simulink model "simulinkmodel"  (R2023a)
settings: Solver=ode4  StartTime=0.0  StopTime=250.0  FixedStep=1e-3  RelTol=1e-3
values from neighbouring files (symbols this model uses):
  ARw = 7.9456    [EOMs_of_AC.m]    (also in constants_simulinkmodel.m)
  b = 9.16    [EOMs_of_AC.m]    (also in constants_simulinkmodel.m)
  c = 1.3333    [EOMs_of_AC.m]    (also in constants_simulinkmodel.m)
  CDf = .005    (= 0.005)    [EOMs_of_AC.m]    (also in constants_simulinkmodel.m)
  CDmint = .002    (= 0.002)    [EOMs_of_AC.m]    (also in constants_simulinkmodel.m)
  CDminvt = .001    (= 0.001)    [EOMs_of_AC.m]    (also in constants_simulinkmodel.m)
  CDminw = .011    (= 0.011)    [EOMs_of_AC.m]    (also in constants_simulinkmodel.m)
  cgt = 3.5    [EOMs_of_AC.m]    (also in constants_simulinkmodel.m)
  cgvt = cgt    (= 3.5)    [EOMs_of_AC.m]    (also in constants_simulinkmodel.m)
  cgw = -.416    (= -0.416)    [EOMs_of_AC.m]    (also in constants_simulinkmodel.m)
  CLat = .76    (= 0.76)    [EOMs_of_AC.m]    (also in constants_simulinkmodel.m)
  CLavt = .0969    (= 0.0969)    [EOMs_of_AC.m]    (also in constants_simulinkmodel.m)
  CLaw = 4.59    [EOMs_of_AC.m]    (also in constants_simulinkmodel.m)
  Clb = -.1    (= -0.1)    [EOMs_of_AC.m]    (also in constants_simulinkmodel.m)
  Clda = 0.244    [EOMs_of_AC.m]    (also in constants_simulinkmodel.m)
  CLow = .421    (= 0.421)    [EOMs_of_AC.m]    (also in constants_simulinkmodel.m)
  Clr = .01    (= 0.01)    [EOMs_of_AC.m]    (also in constants_simulinkmodel.m)
  Cmaf = .114    (= 0.114)    [EOMs_of_AC.m]    (also in constants_simulinkmodel.m)
  Cmw = -0.005    [EOMs_of_AC.m]    (also in constants_simulinkmodel.m)
  Cnda = -0.0128    [EOMs_of_AC.m]    (also in constants_simulinkmodel.m)
  e = .75    (= 0.75)    [EOMs_of_AC.m]    (also in constants_simulinkmodel.m)
  g = 32.17    [EOMs_of_AC.m]    (also in constants_simulinkmodel.m)
  it = 2*d2r    (= 0.0349065850399)    [EOMs_of_AC.m]    (also in constants_simulinkmodel.m = 0.034906585)
  Ixx = 1.9480    (= 1.948)    [EOMs_of_AC.m]    (also in constants_simulinkmodel.m)
  Iyy = 1.5523    [EOMs_of_AC.m]    (also in constants_simulinkmodel.m)
  Izz = 1.9166    [EOMs_of_AC.m]    (also in constants_simulinkmodel.m)
  Kt = .446    (= 0.446)    [EOMs_of_AC.m]    (also in constants_simulinkmodel.m)
  lambda = .72955    (= 0.72955)    [EOMs_of_AC.m]    (also in constants_simulinkmodel.m)
  m = .487669    (= 0.487669)    [EOMs_of_AC.m]    (also in constants_simulinkmodel.m)
  nt = 1    [EOMs_of_AC.m]    (also in constants_simulinkmodel.m)
  nvt = nt    (= 1)    [EOMs_of_AC.m]    (also in constants_simulinkmodel.m)
  rho = .0023081    (= 0.0023081)    [EOMs_of_AC.m]    (also in constants_simulinkmodel.m)
  S = 10.56    [EOMs_of_AC.m]    (also in constants_simulinkmodel.m)
  St = S    (= 10.56)    [EOMs_of_AC.m]    (also in constants_simulinkmodel.m)
  Svt = S    (= 10.56)    [EOMs_of_AC.m]    (also in constants_simulinkmodel.m)
  Te = .422    (= 0.422)    [EOMs_of_AC.m]    (also in constants_simulinkmodel.m)
  Tr = .434    (= 0.434)    [EOMs_of_AC.m]    (also in constants_simulinkmodel.m)
undefined symbols (not defined in the file or in its folder): JSBSim, Rascal110, x_initial
libraries: simulink_extras x12, aerolibfltsims x2, aerolibanimutils x1
(part 1 of 2)
settings Model: Creator=s22734  LastModifiedBy=s22734

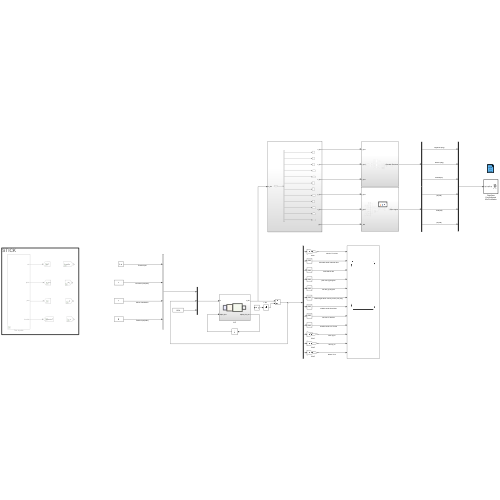
[thumbnail: Simulink's stored preview of the top-level diagram]
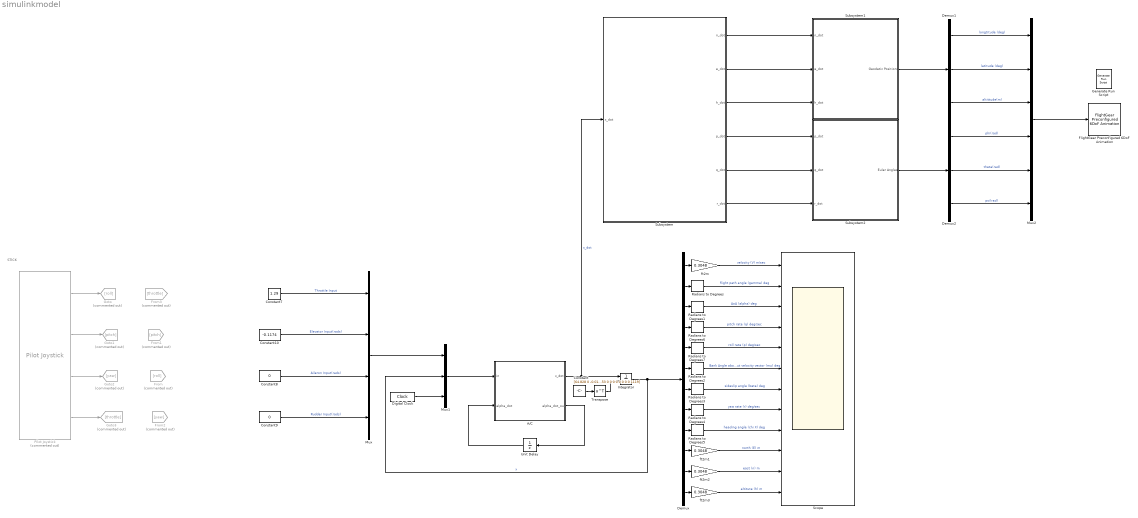
== system simulinkmodel ==
  note: STICK
  A/C : Subsystem
  Constant : Constant  Value=[64.828 0 -0.0153 0 0 0 0 0 0 0 0 1119]  VectorParams1D=off
  Constant10 : Constant  Value=-0.1174
  Constant7 : Constant  Value=1.29
  Constant8 : Constant  Value=0
  Constant9 : Constant  Value=0
  Demux : Demux  Outputs=12
  Demux1 : Demux  Outputs=3
  Demux2 : Demux  Outputs=3
  Digital Clock : DigitalClock
  FlightGear Preconfigured 6DoF Animation : aerolibfltsims/FlightGear Preconfigured 6DoF Animation  xFlightGearVersion=v2019.1  DestinationIpAddress=127.0.0.1  DestinationPort=5502  SampleTime=1/100  packetVersion=24
  From : From  Commented=on  GotoTag=roll
  From1 : From  Commented=on  GotoTag=pitch
  From2 : From  Commented=on  GotoTag=yaw
  From3 : From  Commented=on  GotoTag=throttle
  Generate Run Script : aerolibfltsims/Generate Run Script  Architecture=Win64  dataFlow=Send  GeometryModelName=Rascal110-JSBSim  AirportId=LTAE  RunwayId=21  InitialAltitude=6000  InitialHeading=32  OffsetDistance=0  OffsetAzimuth=0  InstallScenery=on  DisableShaders=off  OriginAddress=127.0.0.1  DestinationPort=5502  OriginPort=5505  LocalAddress=127.0.0.1  OutputFileName=runfg.bat  FlightGearBaseDirectory=C:\FlightGear
  Goto : Goto  Commented=on  GotoTag=roll
  Goto1 : Goto  Commented=on  GotoTag=pitch
  Goto2 : Goto  Commented=on  GotoTag=yaw
  Goto3 : Goto  Commented=on  GotoTag=throttle
  Integrator : Integrator  InitialConditionSource=external  InitialCondition=x_initial
  Mux : Mux
  Mux1 : Mux  Inputs=3
  Mux2 : Mux  Inputs=6
  Pilot Joystick : aerolibanimutils/Pilot Joystick  Commented=on  JoystickID=Joystick1  OutputConfiguration=FourAxis  SampleTime=1/30
  Radians to Degrees{,1..7} (8 alike) : simulink_extras/Transformations/Radians to Degrees
  Scope : Scope  NumInputPorts=12
  Subsystem : Subsystem
  Subsystem1 : Subsystem
  Subsystem2 : Subsystem
  Transpose : Math  Operator=transpose
  Unit Delay : UnitDelay  SampleTime=-1  HasFrameUpgradeWarning=on
  ft2m{,1..3} (4 alike) : Gain  Gain=0.3048
  wires:
  Mux1/1 -> A/C/1(in)
  Constant7/1 -> Mux/1  "Throttle Input"
  Constant10/1 -> Mux/2  "Elevator Input(rads)"
  Constant8/1 -> Mux/3  "Aileron Input(rads)"
  Constant9/1 -> Mux/4  "Rudder Input(rads)"
  Mux/1 -> Mux1/1
  Digital Clock/1 -> Mux1/3
  A/C/1(x_dot) -> Subsystem/1(x_dot), Integrator/1  "x_dot"
  Integrator/1 -> Demux/1, Mux1/2  "x"
  A/C/2(alpha_dot_out) -> Unit Delay/1
  Unit Delay/1 -> A/C/2(alpha_dot)
  Demux/1 -> ft2m/1
  Radians to Degrees/1 -> Scope/2  "flight path angle (gamma) deg"
  Radians to Degrees1/1 -> Scope/3  "AoA (alpha) deg"
  Radians to Degrees6/1 -> Scope/4  "pitch rate (q) deg/sec"
  Radians to Degrees7/1 -> Scope/5  "roll rate (p) deg/sec"
  Radians to Degrees2/1 -> Scope/6  "Bank Angle about velocity vector (mu) deg"
  Radians to Degrees3/1 -> Scope/7  "sideslip angle (beta) deg"
  Radians to Degrees4/1 -> Scope/8  "yaw rate (r) deg/sec"
  Radians to Degrees5/1 -> Scope/9  "heading angle (chi X) deg"
  Demux/10 -> ft2m1/1
  Demux/11 -> ft2m2/1
  Demux/12 -> ft2m3/1
  Constant/1 -> Transpose/1
  Transpose/1 -> Integrator/2
  Demux/2 -> Radians to Degrees/1
  Demux/3 -> Radians to Degrees1/1
  Demux/4 -> Radians to Degrees6/1
  Demux/5 -> Radians to Degrees7/1
  Demux/6 -> Radians to Degrees2/1
  Demux/7 -> Radians to Degrees3/1
  Demux/8 -> Radians to Degrees4/1
  Demux/9 -> Radians to Degrees5/1
  Mux2/1 -> FlightGear Preconfigured 6DoF Animation/1
  Demux1/1 -> Mux2/1  "longtitude (deg)"
  Demux1/2 -> Mux2/2  "latitude (deg)"
  Demux1/3 -> Mux2/3  "altittude(m)"
  Demux2/1 -> Mux2/4  "phi(rad)"
  Demux2/2 -> Mux2/5  "theta(rad)"
  Demux2/3 -> Mux2/6  "psi(rad)"
  Subsystem/1(n_dot) -> Subsystem1/1(n_dot)
  Subsystem/2(e_dot) -> Subsystem1/2(e_dot)
  Subsystem/3(h_dot) -> Subsystem1/3(h_dot)
  Subsystem1/1(Geodetic Positions) -> Demux1/1
  Subsystem/4(p_dot) -> Subsystem2/1(p_dot)
  Subsystem/5(q_dot) -> Subsystem2/2(q_dot)
  Subsystem/6(r_dot) -> Subsystem2/3(r_dot)
  Subsystem2/1(Euler Angles) -> Demux2/1
  ft2m/1 -> Scope/1  "velocity (V) m/sec"
  ft2m3/1 -> Scope/12  "altitute (h) m"
  ft2m2/1 -> Scope/11  "east (n) m"
  ft2m1/1 -> Scope/10  "north (E) m"
  Pilot Joystick/4 -> Goto3/1
  Pilot Joystick/3 -> Goto2/1
  Pilot Joystick/2 -> Goto1/1
  Pilot Joystick/1 -> Goto/1

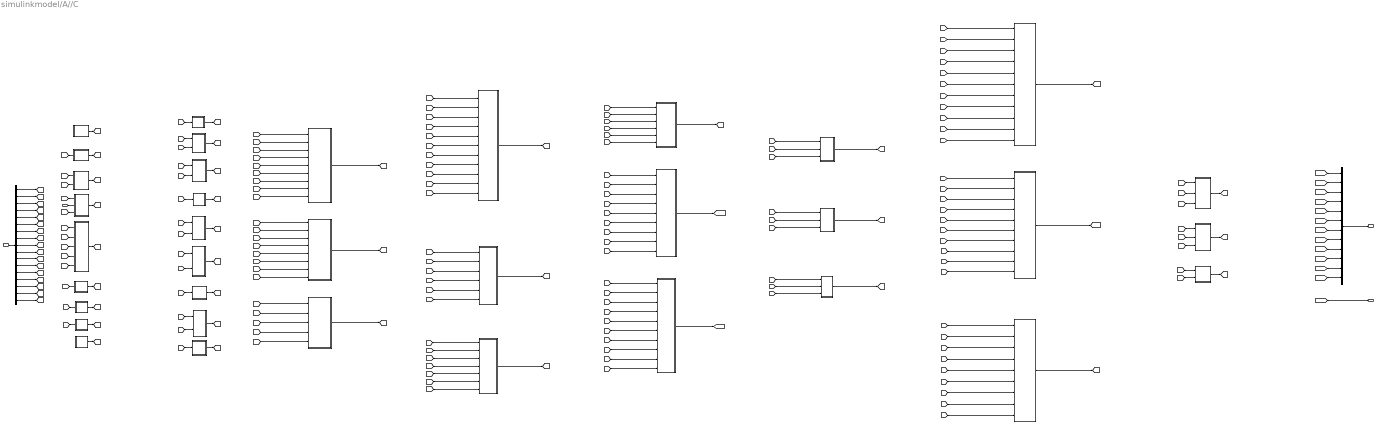
== system simulinkmodel/A//C ==
  note: KINEMATIC EQUATIONS
  note: EOMs
  note: FORCES AND MOMENTS
  note: CONSTANTS
  in : Inport
  alpha_dot : Inport  Port=2
  Demux : Demux  Outputs=17
  Mux : Mux  Inputs=12
  Subsystem : Subsystem
  Subsystem1 : Subsystem
  Subsystem10 : Subsystem
  Subsystem11 : Subsystem
  Subsystem12 : Subsystem
  Subsystem13 : Subsystem
  Subsystem14 : Subsystem
  Subsystem15 : Subsystem
  Subsystem16 : Subsystem
  Subsystem17 : Subsystem
  Subsystem18 : Subsystem
  Subsystem2 : Subsystem
  Subsystem20 : Subsystem
  Subsystem21 : Subsystem
  Subsystem22 : Subsystem
  Subsystem23 : Subsystem
  Subsystem24 : Subsystem
  Subsystem25 : Subsystem
  Subsystem26 : Subsystem
  Subsystem27 : Subsystem
  Subsystem28 : Subsystem
  Subsystem29 : Subsystem
  Subsystem3 : Subsystem
  Subsystem30 : Subsystem
  Subsystem31 : Subsystem
  Subsystem32 : Subsystem
  Subsystem33 : Subsystem
  Subsystem34 : Subsystem
  Subsystem35 : Subsystem
  Subsystem36 : Subsystem
  Subsystem4 : Subsystem
  Subsystem5 : Subsystem
  Subsystem6 : Subsystem
  Subsystem7 : Subsystem
  Subsystem8 : Subsystem
  Subsystem9 : Subsystem
  x_dot : Outport
  alpha_dot_out : Outport  Port=2
  wires:
  in/1 -> Demux/1
  Demux/1 -> [T]
  Demux/2 -> [de]
  Demux/3 -> [drt]
  Demux/4 -> [da]
  Demux/6 -> [gamma]
  Demux/8 -> [q]
  Demux/9 -> [p]
  Demux/10 -> [mu]
  Demux/11 -> [beta]
  Demux/12 -> [r]
  Demux/13 -> [chi]
  Demux/14 -> [north]
  Demux/15 -> [east]
  Demux/17 -> [tm]
  [alpha_dot] -> alpha_dot_out/1
  Mux/1 -> x_dot/1
  [V_dot] -> Mux/1
  [gamma_dot] -> Mux/2
  [alpha_dot] -> Mux/3
  [q_dot] -> Mux/4
  [p_dot] -> Mux/5
  [mu_dot] -> Mux/6
  [beta_dot] -> Mux/7
  [r_dot] -> Mux/8
  [chi_dot] -> Mux/9
  [n_dot] -> Mux/10
  [e_dot] -> Mux/11
  [h_dot] -> Mux/12
  Demux/5 -> [V]
  Demux/16 -> [h]
  Demux/7 -> [alpha]
  Subsystem/1(Kw) -> [Kw]
  [alpha] -> Subsystem20/1(alpha)
  Subsystem20/1(CLw) -> [CLw]
  [Kw] -> Subsystem21/1(Kw)
  [CLw] -> Subsystem21/2(CLw)
  Subsystem21/1(CDw) -> [CDw]
  [V] -> Subsystem22/1(V)
  Subsystem22/1(qb) -> [qb]
  [qb] -> Subsystem23/1(qb)
  [CLw] -> Subsystem23/2(CLw)
  Subsystem23/1(Lw) -> [Lw]
  [qb] -> Subsystem24/1(qb)
  [CDw] -> Subsystem24/2(CDw)
  Subsystem24/1(Dw) -> [Dw]
  [alpha] -> Subsystem25/1(alpha)
  alpha_dot/1 -> Subsystem25/2(alpha_dot)
  [V] -> Subsystem25/3(V)
  Subsystem25/1(E) -> [E]
  [alpha] -> Subsystem2/1(alpha)
  [de] -> Subsystem2/2(de)
  [q] -> Subsystem2/3(q)
  [V] -> Subsystem2/4(V)
  [E] -> Subsystem2/5(E)
  Subsystem2/1(alphat) -> [alphat]
  [alphat] -> Subsystem1/1(alphat)
  Subsystem1/1(CLt) -> [CLt]
  [qb] -> Subsystem26/1(qb)
  Subsystem26/1(Mw) -> [Mw]
  [qb] -> Subsystem27/1(qb)
  Subsystem27/1(Df) -> [Df]
  [qb] -> Subsystem28/1(qb)
  [CLt] -> Subsystem28/2(CLt)
  Subsystem28/1(Lt) -> [Lt]
  [qb] -> Subsystem29/1(qb)
  [CDt] -> Subsystem29/2(CDt)
  Subsystem29/1(Dt) -> [Dt]
  [qb] -> Subsystem30/1(qb)
  [Cmf] -> Subsystem30/2(Cmf)
  Subsystem30/1(Mf) -> [Mf]
  [qb] -> Subsystem31/1(qb)
  Subsystem31/1(Dvt) -> [Dvt]
  Subsystem32/1(Clp) -> [Clp]
  [alpha] -> Subsystem33/1(alpha)
  Subsystem33/1(Cmf) -> [Cmf]
  [CLt] -> Subsystem34/1(CLt)
  Subsystem34/1(CDt) -> [CDt]
  [Lw] -> Subsystem35/1(Lw)
  [Lt] -> Subsystem35/2(Lt)
  [E] -> Subsystem35/3(E)
  [q] -> Subsystem35/4(q)
  [V] -> Subsystem35/5(V)
  [Dt] -> Subsystem35/6(Dt)
  [Dvt] -> Subsystem35/7(Dvt)
  [q] -> Subsystem35/8(In9)
  [V] -> Subsystem35/9(In10)
  Subsystem35/1(L) -> [L]
  [Dw] -> Subsystem3/1(Dw)
  [Lt] -> Subsystem3/3(Lt)
  [Dt] -> Subsystem3/4(Dt)
  [Dvt] -> Subsystem3/5(Dvt)
  [E] -> Subsystem3/6(E)
  [q] -> Subsystem3/7(q)
  [V] -> Subsystem3/8(V)
  Subsystem3/1(D) -> [D]
  [qb] -> Subsystem4/1(qb)
  [beta] -> Subsystem4/2(beta)
  [drt] -> Subsystem4/3(drt)
  [r] -> Subsystem4/4(r)
  [V] -> Subsystem4/5(V)
  Subsystem4/1(Y) -> [Y]
  [Df] -> Subsystem3/2(Df)
  [Lw] -> Subsystem5/1(Lw)
  [alpha] -> Subsystem5/2(alpha)
  [Dw] -> Subsystem5/3(Dw)
  [Mw] -> Subsystem5/4(Mw)
  [Lt] -> Subsystem5/5(Lt)
  [E] -> Subsystem5/6(E)
  [q] -> Subsystem5/7(q)
  [V] -> Subsystem5/8(V)
  [Dt] -> Subsystem5/9(Dt)
  [Dvt] -> Subsystem5/10(Dvt)
  [Mf] -> Subsystem5/11(Mf)
  Subsystem5/1(Mc) -> [Mc]
  [qb] -> Subsystem6/1(qb)
  [beta] -> Subsystem6/2(beta)
  [drt] -> Subsystem6/3(drt)
  [r] -> Subsystem6/4(r)
  [V] -> Subsystem6/5(V)
  [da] -> Subsystem6/6(da)
  Subsystem6/1(Nc) -> [Nc]
  [qb] -> Subsystem7/1(qb)
  [Clp] -> Subsystem7/2(Clp)
  [p] -> Subsystem7/3(p)
  [V] -> Subsystem7/4(V)
  [beta] -> Subsystem7/5(beta)
  [drt] -> Subsystem7/6(drt)
  [da] -> Subsystem7/7(da)
  Subsystem7/1(Lc) -> [Lc]
  [D] -> Subsystem8/1(D)
  [beta] -> Subsystem8/2(beta)
  [Y] -> Subsystem8/3(Y)
  [T] -> Subsystem8/4(T)
  [alpha] -> Subsystem8/5(alpha)
  [gamma] -> Subsystem8/6(gamma)
  Subsystem8/1(V_dot) -> [V_dot]
  [D] -> Subsystem9/1(D)
  [beta] -> Subsystem9/2(beta)
  [mu] -> Subsystem9/3(mu)
  [Y] -> Subsystem9/4(Y)
  [L] -> Subsystem9/5(L)
  [T] -> Subsystem9/6(T)
  [alpha] -> Subsystem9/7(alpha)
  [V] -> Subsystem9/8(V)
  [gamma] -> Subsystem9/9(gamma)
  Subsystem9/1(gamma_dot) -> [gamma_dot]
  [q] -> Subsystem10/1(q)
  [p] -> Subsystem10/2(p)
  [alpha] -> Subsystem10/3(alpha)
  [r] -> Subsystem10/4(r)
  [beta] -> Subsystem10/5(beta)
  [L] -> Subsystem10/6(L)
  [T] -> Subsystem10/7(T)
  [V] -> Subsystem10/8(V)
  [gamma] -> Subsystem10/9(gamma)
  [mu] -> Subsystem10/10(mu)
  Subsystem10/1(alpha_dot) -> [alpha_dot]
  [Mc] -> Subsystem11/1(Mc)
  [p] -> Subsystem11/2(p)
  [r] -> Subsystem11/3(r)
  Subsystem11/1(q_dot) -> [q_dot]
  [Lc] -> Subsystem12/1(Lc)
  [q] -> Subsystem12/2(q)
  [r] -> Subsystem12/3(r)
  Subsystem12/1(p_dot) -> [p_dot]
  [Nc] -> Subsystem13/1(Nc)
  [p] -> Subsystem13/2(p)
  [q] -> Subsystem13/3(q)
  Subsystem13/1(r_dot) -> [r_dot]
  [p] -> Subsystem14/1(p)
  [alpha] -> Subsystem14/2(alpha)
  [r] -> Subsystem14/3(r)
  [beta] -> Subsystem14/4(beta)
  [D] -> Subsystem14/5(D)
  [mu] -> Subsystem14/6(mu)
  [gamma] -> Subsystem14/7(gamma)
  [Y] -> Subsystem14/8(Y)
  [L] -> Subsystem14/9(L)
  [T] -> Subsystem14/10(T)
  [V] -> Subsystem14/11(V)
  Subsystem14/1(mu_dot) -> [mu_dot]
  [r] -> Subsystem15/1(r)
  [alpha] -> Subsystem15/2(alpha)
  [p] -> Subsystem15/3(p)
  [D] -> Subsystem15/4(D)
  [beta] -> Subsystem15/5(beta)
  [Y] -> Subsystem15/6(Y)
  [T] -> Subsystem15/7(T)
  [V] -> Subsystem15/8(V)
  [gamma] -> Subsystem15/9(gamma)
  [mu] -> Subsystem15/10(mu)
  Subsystem15/1(beta_dot) -> [beta_dot]
  [V] -> Subsystem16/1(V)
  [gamma] -> Subsystem16/2(gamma)
  [chi] -> Subsystem16/3(chi)
  Subsystem16/1(n_dot) -> [n_dot]
  [V] -> Subsystem17/1(V)
  [gamma] -> Subsystem17/2(gamma)
  [chi] -> Subsystem17/3(chi)
  Subsystem17/1(e_dot) -> [e_dot]
  [V] -> Subsystem18/1(V)
  [gamma] -> Subsystem18/2(gamma)
  Subsystem18/1(h_dot) -> [h_dot]
  [D] -> Subsystem36/1(D)
  [beta] -> Subsystem36/2(beta)
  [mu] -> Subsystem36/3(mu)
  [Y] -> Subsystem36/4(Y)
  [L] -> Subsystem36/5(L)
  [T] -> Subsystem36/6(T)
  [alpha] -> Subsystem36/7(alpha)
  [V] -> Subsystem36/8(V)
  [gamma] -> Subsystem36/9(gamma)
  Subsystem36/1(chi_dot) -> [chi_dot]

== system simulinkmodel/Subsystem ==
  x_dot : Inport
  Demux1 : Demux  Outputs=12
  Terminator{,1..5} (6 alike) : Terminator
  n_dot : Outport
  e_dot : Outport  Port=2
  h_dot : Outport  Port=3
  p_dot : Outport  Port=4
  q_dot : Outport  Port=5
  r_dot : Outport  Port=6
  wires:
  Demux1/12 -> h_dot/1  "h_dot"
  Demux1/9 -> Terminator5/1  "chi_dot"
  Demux1/7 -> Terminator4/1  "beta_dot"
  x_dot/1 -> Demux1/1
  Demux1/5 -> p_dot/1  "p_dot"
  Demux1/10 -> n_dot/1  "n_dot"
  Demux1/11 -> e_dot/1  "e_dot"
  Demux1/8 -> r_dot/1  "r_dot"
  Demux1/4 -> q_dot/1  "q_dot"
  Demux1/3 -> Terminator2/1  "alpha_dot"
  Demux1/6 -> Terminator3/1  "mu_dot"
  Demux1/2 -> Terminator1/1  "gamma_dot"
  Demux1/1 -> Terminator/1  "V_dot"

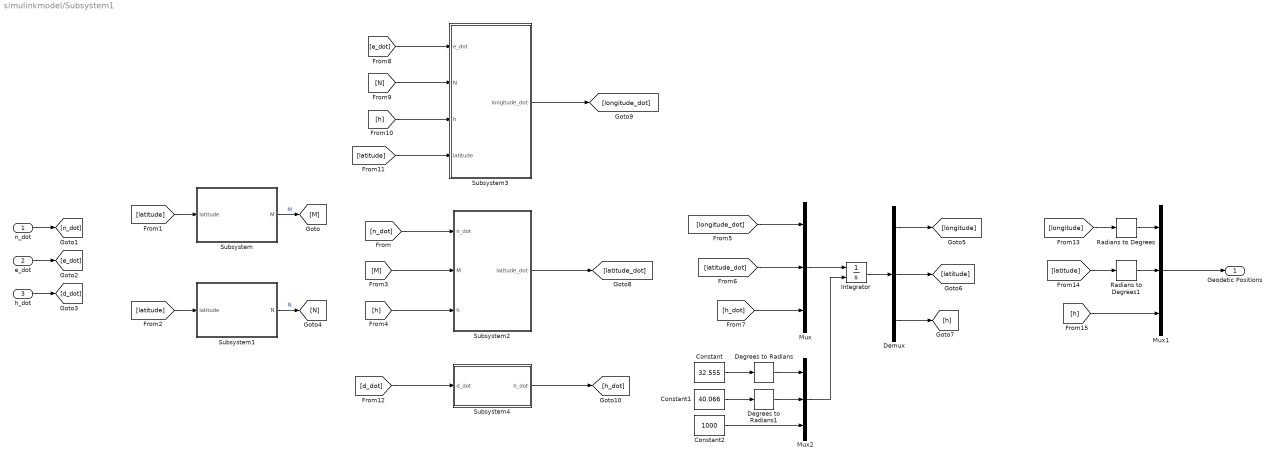
== system simulinkmodel/Subsystem1 ==
  n_dot : Inport
  e_dot : Inport  Port=2
  h_dot : Inport  Port=3
  Constant : Constant  Value=32.555
  Constant1 : Constant  Value=40.066
  Constant2 : Constant  Value=1000
  Degrees to Radians : simulink_extras/Transformations/Degrees to Radians
  Degrees to Radians1 : simulink_extras/Transformations/Degrees to Radians
  Demux : Demux  Outputs=3
  Integrator : Integrator  InitialConditionSource=external  InitialCondition=[32.555;40.066;3000]
  Mux : Mux  Inputs=3
  Mux1 : Mux  Inputs=3
  Mux2 : Mux  Inputs=3
  Radians to Degrees : simulink_extras/Transformations/Radians to Degrees
  Radians to Degrees1 : simulink_extras/Transformations/Radians to Degrees
  Subsystem : Subsystem
  Subsystem1 : Subsystem
  Subsystem2 : Subsystem
  Subsystem3 : Subsystem
  Subsystem4 : Subsystem
  Geodetic Positions : Outport
  wires:
  e_dot/1 -> [e_dot]
  n_dot/1 -> [n_dot]
  h_dot/1 -> [d_dot]
  [latitude] -> Subsystem/1(latitude)
  Subsystem/1(M) -> [M]  "M"
  [latitude] -> Subsystem1/1(latitude)
  Subsystem1/1(N) -> [N]  "N"
  [longitude_dot] -> Mux/1
  [latitude_dot] -> Mux/2
  [h_dot] -> Mux/3
  Mux/1 -> Integrator/1
  Integrator/1 -> Demux/1
  Demux/1 -> [longitude]
  Demux/3 -> [h]
  Demux/2 -> [latitude]
  [n_dot] -> Subsystem2/1(n_dot)
  [M] -> Subsystem2/2(M)
  [h] -> Subsystem2/3(h)
  Subsystem2/1(latitude_dot) -> [latitude_dot]
  [e_dot] -> Subsystem3/1(e_dot)
  [N] -> Subsystem3/2(N)
  [h] -> Subsystem3/3(h)
  [latitude] -> Subsystem3/4(latitude)
  Subsystem3/1(longitude_dot) -> [longitude_dot]
  [d_dot] -> Subsystem4/1(d_dot)
  Subsystem4/1(h_dot) -> [h_dot]
  Mux1/1 -> Geodetic Positions/1
  [longitude] -> Radians to Degrees/1
  [latitude] -> Radians to Degrees1/1
  [h] -> Mux1/3
  Radians to Degrees1/1 -> Mux1/2
  Radians to Degrees/1 -> Mux1/1
  Constant/1 -> Degrees to Radians/1
  Degrees to Radians/1 -> Mux2/1
  Constant1/1 -> Degrees to Radians1/1
  Degrees to Radians1/1 -> Mux2/2
  Constant2/1 -> Mux2/3
  Mux2/1 -> Integrator/2

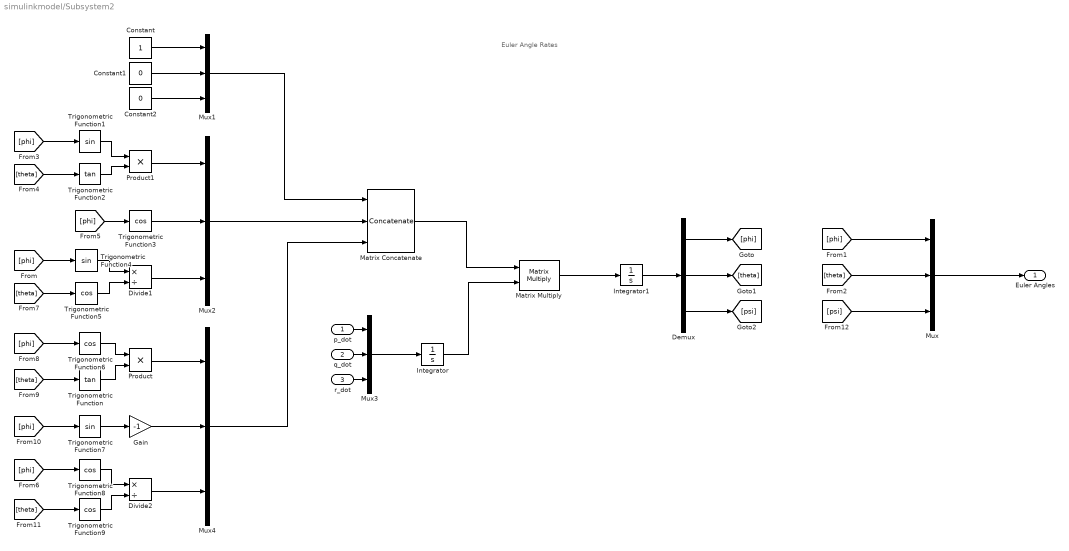
== system simulinkmodel/Subsystem2 ==
  note: Euler Angle Rates
  p_dot : Inport
  q_dot : Inport  Port=2
  r_dot : Inport  Port=3
  Constant : Constant
  Constant1 : Constant  Value=0
  Constant2 : Constant  Value=0
  Demux : Demux  Outputs=3
  Divide1 : Product  Inputs=*/
  Divide2 : Product  Inputs=*/
  Gain : Gain  Gain=-1
  Integrator : Integrator  InitialCondition=[0;0;0]
  Integrator1 : Integrator  InitialCondition=[0;0;0]
  Matrix Concatenate : Concatenate  NumInputs=3  Mode=Multidimensional array  ConcatenateDimension=2
  Matrix Multiply : Product  Multiplication=Matrix(*)
  Mux{,1..4} (5 alike) : Mux  Inputs=3
  Product : Product
  Product1 : Product
  Trigonometric Function : Trigonometry  Operator=tan
  Trigonometric Function1 : Trigonometry
  Trigonometric Function2 : Trigonometry  Operator=tan
  Trigonometric Function{3,5..6,8..9} (5 alike) : Trigonometry  Operator=cos
  Trigonometric Function4 : Trigonometry
  Trigonometric Function7 : Trigonometry
  Euler Angles : Outport
  wires:
  q_dot/1 -> Mux3/2
  Matrix Multiply/1 -> Integrator1/1
  p_dot/1 -> Mux3/1
  Mux3/1 -> Integrator/1
  r_dot/1 -> Mux3/3
  Integrator/1 -> Matrix Multiply/2
  Integrator1/1 -> Demux/1
  Demux/1 -> [phi]
  Demux/2 -> [theta]
  Demux/3 -> [psi]
  Constant/1 -> Mux1/1
  Constant1/1 -> Mux1/2
  Constant2/1 -> Mux1/3
  [phi] -> Trigonometric Function1/1
  Trigonometric Function1/1 -> Product1/1
  [theta] -> Trigonometric Function2/1
  Trigonometric Function2/1 -> Product1/2
  Product1/1 -> Mux2/1
  [phi] -> Trigonometric Function3/1
  Trigonometric Function3/1 -> Mux2/2
  Trigonometric Function4/1 -> Divide1/1
  [phi] -> Trigonometric Function4/1
  [theta] -> Trigonometric Function5/1
  Trigonometric Function5/1 -> Divide1/2
  Divide1/1 -> Mux2/3
  [phi] -> Trigonometric Function6/1
  [theta] -> Trigonometric Function/1
  Trigonometric Function6/1 -> Product/1
  Trigonometric Function/1 -> Product/2
  Product/1 -> Mux4/1
  Trigonometric Function7/1 -> Gain/1
  [phi] -> Trigonometric Function7/1
  Gain/1 -> Mux4/2
  [theta] -> Trigonometric Function9/1
  [phi] -> Trigonometric Function8/1
  Trigonometric Function8/1 -> Divide2/1
  Trigonometric Function9/1 -> Divide2/2
  Divide2/1 -> Mux4/3
  Mux1/1 -> Matrix Concatenate/1
  Mux2/1 -> Matrix Concatenate/2
  Mux4/1 -> Matrix Concatenate/3
  Matrix Concatenate/1 -> Matrix Multiply/1
  [psi] -> Mux/3
  [theta] -> Mux/2
  [phi] -> Mux/1
  Mux/1 -> Euler Angles/1

== system simulinkmodel/A//C/Subsystem ==
  note: Induced Drag Coefficient
  Constant3 : Constant
  Constant4 : Constant  Value=ARw
  Constant5 : Constant  Value=e
  Divide : Product  Inputs=*/
  Pi : Constant  Value=pi  OutDataTypeStr=Inherit: Inherit via back propagation
  Product1 : Product  Inputs=3
  Kw : Outport
  wires:
  Constant5/1 -> Product1/3
  Product1/1 -> Divide/2
  Pi/1 -> Product1/1
  Constant3/1 -> Divide/1
  Constant4/1 -> Product1/2
  Divide/1 -> Kw/1

== system simulinkmodel/A//C/Subsystem1 ==
  note: Tail Lift Coefficient
  alphat : Inport
  Constant15 : Constant  Value=CLat
  Product6 : Product
  CLt : Outport
  wires:
  alphat/1 -> Product6/2
  Constant15/1 -> Product6/1
  Product6/1 -> CLt/1

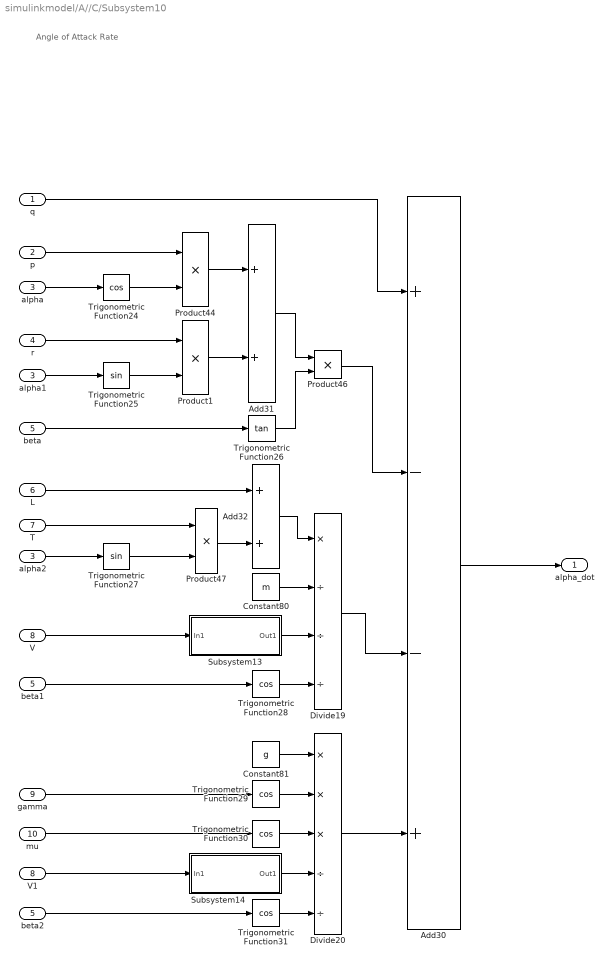
== system simulinkmodel/A//C/Subsystem10 ==
  note: Angle of Attack Rate
  q : Inport
  p : Inport  Port=2
  alpha : Inport  Port=3
  r : Inport  Port=4
  beta : Inport  Port=5
  L : Inport  Port=6
  T : Inport  Port=7
  V : Inport  Port=8
  gamma : Inport  Port=9
  mu : Inport  Port=10
  Add30 : Sum  Inputs=+--+
  Add31 : Sum
  Add32 : Sum
  Constant80 : Constant  Value=m
  Constant81 : Constant  Value=g
  Divide19 : Product  Inputs=*///
  Divide20 : Product  Inputs=***//
  Product{1,44,46..47} (4 alike) : Product
  Subsystem13 : Subsystem
  Subsystem14 : Subsystem
  Trigonometric Function{24,28..31} (5 alike) : Trigonometry  Operator=cos
  Trigonometric Function25 : Trigonometry
  Trigonometric Function26 : Trigonometry  Operator=tan
  Trigonometric Function27 : Trigonometry
  V1 : InportShadow  Port=8
  alpha1 : InportShadow  Port=3
  alpha2 : InportShadow  Port=3
  beta1 : InportShadow  Port=5
  beta2 : InportShadow  Port=5
  alpha_dot : Outport
  wires:
  Add31/1 -> Product46/1
  r/1 -> Product1/1
  Product1/1 -> Add31/2
  Trigonometric Function29/1 -> Divide20/2
  Trigonometric Function24/1 -> Product44/2
  Trigonometric Function28/1 -> Divide19/4
  mu/1 -> Trigonometric Function30/1
  Trigonometric Function31/1 -> Divide20/5
  Subsystem13/1(Out1) -> Divide19/3
  Trigonometric Function25/1 -> Product1/2
  Constant81/1 -> Divide20/1
  Constant80/1 -> Divide19/2
  Product44/1 -> Add31/1
  Trigonometric Function26/1 -> Product46/2
  Trigonometric Function30/1 -> Divide20/3
  gamma/1 -> Trigonometric Function29/1
  L/1 -> Add32/1
  beta/1 -> Trigonometric Function26/1
  Add32/1 -> Divide19/1
  Subsystem14/1(Out1) -> Divide20/4
  Divide20/1 -> Add30/4
  Divide19/1 -> Add30/3
  Product47/1 -> Add32/2
  Trigonometric Function27/1 -> Product47/2
  Product46/1 -> Add30/2
  q/1 -> Add30/1
  alpha2/1 -> Trigonometric Function27/1
  alpha/1 -> Trigonometric Function24/1
  beta2/1 -> Trigonometric Function31/1
  p/1 -> Product44/1
  Add30/1 -> alpha_dot/1
  V1/1 -> Subsystem14/1(In1)
  alpha1/1 -> Trigonometric Function25/1
  T/1 -> Product47/1
  V/1 -> Subsystem13/1(In1)
  beta1/1 -> Trigonometric Function28/1

== system simulinkmodel/A//C/Subsystem11 ==
  note: Pitch Rate Derivative
  Mc : Inport
  p : Inport  Port=2
  r : Inport  Port=3
  Add33 : Sum
  Add34 : Sum  Inputs=+-
  Constant82 : Constant  Value=Iyy
  Constant83 : Constant  Value=Izz
  Constant84 : Constant  Value=Ixx
  Constant85 : Constant  Value=Iyy
  Divide21 : Product  Inputs=*/
  Divide22 : Product  Inputs=*/
  Product48 : Product  Inputs=3
  Product49 : Product  Inputs=3
  p1 : InportShadow  Port=2
  r1 : InportShadow  Port=3
  q_dot : Outport
  wires:
  Constant82/1 -> Divide21/2
  Product48/1 -> Add34/1
  Divide21/1 -> Add33/1
  Constant85/1 -> Divide22/2
  Divide22/1 -> Add33/2
  Add34/1 -> Divide22/1
  r1/1 -> Product49/3
  p/1 -> Product48/2
  Constant84/1 -> Product49/1
  Constant83/1 -> Product48/1
  Product49/1 -> Add34/2
  Add33/1 -> q_dot/1
  Mc/1 -> Divide21/1
  r/1 -> Product48/3
  p1/1 -> Product49/2

== system simulinkmodel/A//C/Subsystem12 ==
  note: Roll Rate Derivative
  Lc : Inport
  q : Inport  Port=2
  r : Inport  Port=3
  Add35 : Sum  Inputs=+-
  Add36 : Sum
  Constant86 : Constant  Value=Ixx
  Constant87 : Constant  Value=Iyy
  Constant88 : Constant  Value=Izz
  Constant89 : Constant  Value=Ixx
  Divide23 : Product  Inputs=*/
  Divide24 : Product  Inputs=*/
  Product50 : Product  Inputs=3
  Product51 : Product  Inputs=3
  q1 : InportShadow  Port=2
  r1 : InportShadow  Port=3
  p_dot : Outport
  wires:
  Product50/1 -> Add35/1
  Add35/1 -> Divide24/1
  Constant87/1 -> Product50/1
  Constant89/1 -> Divide24/2
  Constant88/1 -> Product51/1
  Divide24/1 -> Add36/2
  Divide23/1 -> Add36/1
  Product51/1 -> Add35/2
  Constant86/1 -> Divide23/2
  Lc/1 -> Divide23/1
  q/1 -> Product50/2
  r/1 -> Product50/3
  r1/1 -> Product51/3
  Add36/1 -> p_dot/1
  q1/1 -> Product51/2

== system simulinkmodel/A//C/Subsystem13 ==
  note: Yaw Rate Derivative
  Nc : Inport
  p : Inport  Port=2
  q : Inport  Port=3
  Add44 : Sum
  Add45 : Sum  Inputs=+-
  Constant94 : Constant  Value=Izz
  Constant95 : Constant  Value=Ixx
  Constant96 : Constant  Value=Iyy
  Constant97 : Constant  Value=Izz
  Divide30 : Product  Inputs=*/
  Divide31 : Product  Inputs=*/
  Product67 : Product  Inputs=3
  Product68 : Product  Inputs=3
  p1 : InportShadow  Port=2
  q1 : InportShadow  Port=3
  r_dot : Outport
  wires:
  Divide31/1 -> Add44/2
  Constant97/1 -> Divide31/2
  Constant94/1 -> Divide30/2
  Divide30/1 -> Add44/1
  Product68/1 -> Add45/2
  Add45/1 -> Divide31/1
  Product67/1 -> Add45/1
  Constant96/1 -> Product68/1
  Constant95/1 -> Product67/1
  p1/1 -> Product68/2
  Add44/1 -> r_dot/1
  q/1 -> Product67/3
  q1/1 -> Product68/3
  p/1 -> Product67/2
  Nc/1 -> Divide30/1

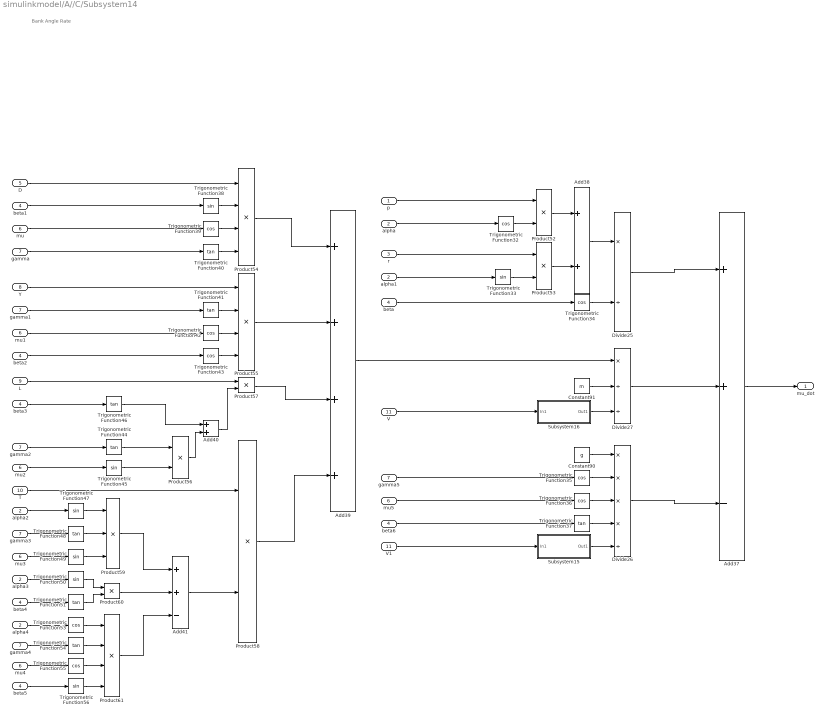
== system simulinkmodel/A//C/Subsystem14 ==
  note: Bank Angle Rate
  p : Inport
  alpha : Inport  Port=2
  r : Inport  Port=3
  beta : Inport  Port=4
  D : Inport  Port=5
  mu : Inport  Port=6
  gamma : Inport  Port=7
  Y : Inport  Port=8
  L : Inport  Port=9
  T : Inport  Port=10
  V : Inport  Port=11
  Add37 : Sum  Inputs=++-
  Add38 : Sum
  Add39 : Sum  Inputs=++++
  Add40 : Sum
  Add41 : Sum  Inputs=++-
  Constant90 : Constant  Value=g
  Constant91 : Constant  Value=m
  Divide25 : Product  Inputs=*/
  Divide26 : Product  Inputs=****/
  Divide27 : Product  Inputs=*//
  Product{52..53,56..58,60} (6 alike) : Product
  Product54 : Product  Inputs=4
  Product55 : Product  Inputs=4
  Product59 : Product  Inputs=3
  Product61 : Product  Inputs=4
  Subsystem15 : Subsystem
  Subsystem16 : Subsystem
  Trigonometric Function{32,34..36,39,42..43,53,55} (9 alike) : Trigonometry  Operator=cos
  Trigonometric Function{33,38,45,47,49..50,56} (7 alike) : Trigonometry
  Trigonometric Function{37,40..41,44,46,48,51,54} (8 alike) : Trigonometry  Operator=tan
  V1 : InportShadow  Port=11
  alpha{1..4} (4 alike) : InportShadow  Port=2
  beta{1..6} (6 alike) : InportShadow  Port=4
  gamma{1..5} (5 alike) : InportShadow  Port=7
  mu{1..5} (5 alike) : InportShadow  Port=6
  mu_dot : Outport
  wires:
  beta1/1 -> Trigonometric Function38/1
  Trigonometric Function54/1 -> Product61/2
  Divide26/1 -> Add37/3
  Product58/1 -> Add39/4
  Trigonometric Function39/1 -> Product54/3
  Product57/1 -> Add39/3
  Trigonometric Function33/1 -> Product53/2
  beta6/1 -> Trigonometric Function37/1
  Trigonometric Function32/1 -> Product52/2
  Constant90/1 -> Divide26/1
  alpha/1 -> Trigonometric Function32/1
  Trigonometric Function48/1 -> Product59/2
  gamma5/1 -> Trigonometric Function35/1
  Trigonometric Function47/1 -> Product59/1
  Divide25/1 -> Add37/1
  Product52/1 -> Add38/1
  Product53/1 -> Add38/2
  Divide27/1 -> Add37/2
  Product59/1 -> Add41/1
  Trigonometric Function53/1 -> Product61/1
  Add40/1 -> Product57/2
  Trigonometric Function56/1 -> Product61/4
  Add39/1 -> Divide27/1
  Trigonometric Function38/1 -> Product54/2
  Trigonometric Function41/1 -> Product55/2
  r/1 -> Product53/1
  V/1 -> Subsystem16/1(In1)
  p/1 -> Product52/1
  Trigonometric Function34/1 -> Divide25/2
  Product56/1 -> Add40/2
  Add38/1 -> Divide25/1
  Subsystem15/1(Out1) -> Divide26/5
  Trigonometric Function36/1 -> Divide26/3
  Trigonometric Function45/1 -> Product56/2
  Trigonometric Function50/1 -> Product60/1
  Trigonometric Function37/1 -> Divide26/4
  Constant91/1 -> Divide27/2
  Subsystem16/1(Out1) -> Divide27/3
  beta5/1 -> Trigonometric Function56/1
  Trigonometric Function49/1 -> Product59/3
  Trigonometric Function44/1 -> Product56/1
  Trigonometric Function55/1 -> Product61/3
  Trigonometric Function46/1 -> Add40/1
  Trigonometric Function35/1 -> Divide26/2
  beta2/1 -> Trigonometric Function43/1
  Product60/1 -> Add41/2
  Product61/1 -> Add41/3
  Trigonometric Function40/1 -> Product54/4
  gamma2/1 -> Trigonometric Function44/1
  Product55/1 -> Add39/2
  V1/1 -> Subsystem15/1(In1)
  mu2/1 -> Trigonometric Function45/1
  Trigonometric Function42/1 -> Product55/3
  Trigonometric Function51/1 -> Product60/2
  Trigonometric Function43/1 -> Product55/4
  Y/1 -> Product55/1
  mu3/1 -> Trigonometric Function49/1
  Product54/1 -> Add39/1
  Add41/1 -> Product58/2
  gamma/1 -> Trigonometric Function40/1
  mu1/1 -> Trigonometric Function42/1
  mu5/1 -> Trigonometric Function36/1
  alpha1/1 -> Trigonometric Function33/1
  D/1 -> Product54/1
  mu/1 -> Trigonometric Function39/1
  T/1 -> Product58/1
  beta/1 -> Trigonometric Function34/1
  Add37/1 -> mu_dot/1
  mu4/1 -> Trigonometric Function55/1
  L/1 -> Product57/1
  gamma3/1 -> Trigonometric Function48/1
  alpha2/1 -> Trigonometric Function47/1
  beta3/1 -> Trigonometric Function46/1
  gamma4/1 -> Trigonometric Function54/1
  alpha4/1 -> Trigonometric Function53/1
  alpha3/1 -> Trigonometric Function50/1
  gamma1/1 -> Trigonometric Function41/1
  beta4/1 -> Trigonometric Function51/1

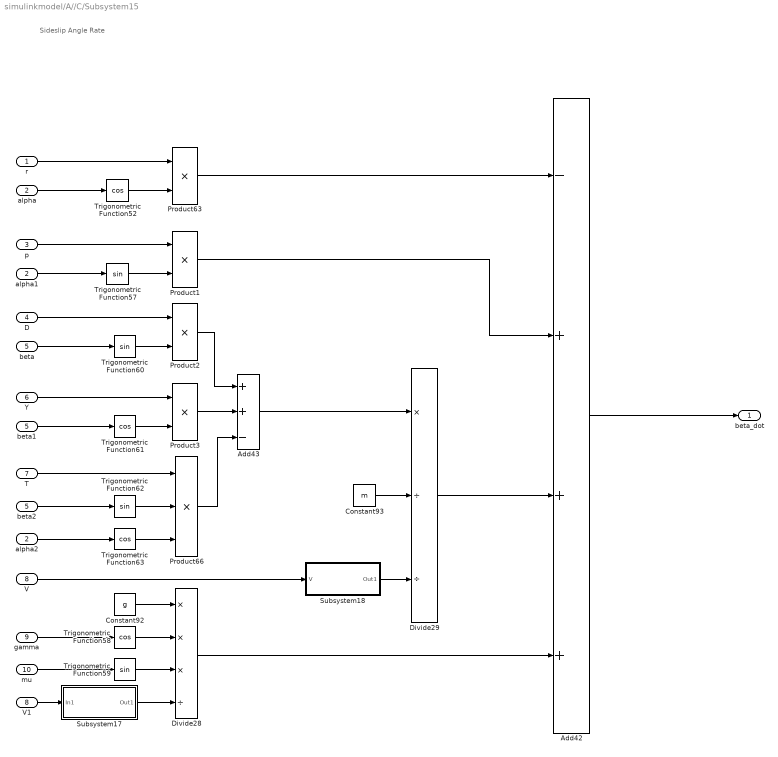
== system simulinkmodel/A//C/Subsystem15 ==
  note: Sideslip Angle Rate
  r : Inport
  alpha : Inport  Port=2
  p : Inport  Port=3
  D : Inport  Port=4
  beta : Inport  Port=5
  Y : Inport  Port=6
  T : Inport  Port=7
  V : Inport  Port=8
  gamma : Inport  Port=9
  mu : Inport  Port=10
  Add42 : Sum  Inputs=-+++
  Add43 : Sum  Inputs=++-
  Constant92 : Constant  Value=g
  Constant93 : Constant  Value=m
  Divide28 : Product  Inputs=***/
  Divide29 : Product  Inputs=*//
  Product{1..3,63} (4 alike) : Product
  Product66 : Product  Inputs=3
  Subsystem17 : Subsystem
  Subsystem18 : Subsystem
  Trigonometric Function{52,58,61,63} (4 alike) : Trigonometry  Operator=cos
  Trigonometric Function{57,59..60,62} (4 alike) : Trigonometry
  V1 : InportShadow  Port=8
  alpha1 : InportShadow  Port=2
  alpha2 : InportShadow  Port=2
  beta1 : InportShadow  Port=5
  beta2 : InportShadow  Port=5
  beta_dot : Outport
  wires:
  mu/1 -> Trigonometric Function59/1
  Divide29/1 -> Add42/3
  gamma/1 -> Trigonometric Function58/1
  Trigonometric Function63/1 -> Product66/3
  p/1 -> Product1/1
  Product2/1 -> Add43/1
  Product66/1 -> Add43/3
  V1/1 -> Subsystem17/1(In1)
  Trigonometric Function60/1 -> Product2/2
  Subsystem17/1(Out1) -> Divide28/4
  Trigonometric Function61/1 -> Product3/2
  Divide28/1 -> Add42/4
  Constant93/1 -> Divide29/2
  Trigonometric Function59/1 -> Divide28/3
  alpha/1 -> Trigonometric Function52/1
  V/1 -> Subsystem18/1(V)
  Trigonometric Function62/1 -> Product66/2
  Add43/1 -> Divide29/1
  Product1/1 -> Add42/2
  alpha2/1 -> Trigonometric Function63/1
  Trigonometric Function52/1 -> Product63/2
  Trigonometric Function58/1 -> Divide28/2
  Product63/1 -> Add42/1
  Subsystem18/1(Out1) -> Divide29/3
  Add42/1 -> beta_dot/1
  beta1/1 -> Trigonometric Function61/1
  Constant92/1 -> Divide28/1
  Trigonometric Function57/1 -> Product1/2
  Product3/1 -> Add43/2
  r/1 -> Product63/1
  alpha1/1 -> Trigonometric Function57/1
  beta/1 -> Trigonometric Function60/1
  T/1 -> Product66/1
  Y/1 -> Product3/1
  beta2/1 -> Trigonometric Function62/1
  D/1 -> Product2/1

== system simulinkmodel/A//C/Subsystem16 ==
  note: North Position Rate
  V : Inport
  gamma : Inport  Port=2
  chi : Inport  Port=3
  Product75 : Product  Inputs=3
  Trigonometric Function75 : Trigonometry  Operator=cos
  Trigonometric Function76 : Trigonometry  Operator=cos
  n_dot : Outport
  wires:
  Trigonometric Function76/1 -> Product75/3
  Trigonometric Function75/1 -> Product75/2
  chi/1 -> Trigonometric Function76/1
  V/1 -> Product75/1
  Product75/1 -> n_dot/1
  gamma/1 -> Trigonometric Function75/1

== system simulinkmodel/A//C/Subsystem17 ==
  note: East Position Rate
  V : Inport
  gamma : Inport  Port=2
  chi : Inport  Port=3
  Product76 : Product  Inputs=3
  Trigonometric Function77 : Trigonometry  Operator=cos
  Trigonometric Function78 : Trigonometry
  e_dot : Outport
  wires:
  Trigonometric Function77/1 -> Product76/2
  gamma/1 -> Trigonometric Function77/1
  Trigonometric Function78/1 -> Product76/3
  V/1 -> Product76/1
  Product76/1 -> e_dot/1
  chi/1 -> Trigonometric Function78/1

== system simulinkmodel/A//C/Subsystem18 ==
  note: Altitude Rate
  V : Inport
  gamma : Inport  Port=2
  Product77 : Product
  Trigonometric Function79 : Trigonometry
  h_dot : Outport
  wires:
  Trigonometric Function79/1 -> Product77/2
  Product77/1 -> h_dot/1
  gamma/1 -> Trigonometric Function79/1
  V/1 -> Product77/1

== system simulinkmodel/A//C/Subsystem2 ==
  note: AoA of Tail
  alpha : Inport
  de : Inport  Port=2
  q : Inport  Port=3
  V : Inport  Port=4
  E : Inport  Port=5
  Add5 : Sum  Inputs=++++-
  Constant12 : Constant  Value=it
  Constant13 : Constant  Value=cgt
  Constant14 : Constant  Value=Te
  Divide3 : Product  Inputs=**/
  Product5 : Product
  Subsystem1 : Subsystem
  alphat : Outport
  wires:
  Add5/1 -> alphat/1
  de/1 -> Product5/1
  Constant13/1 -> Divide3/2
  Divide3/1 -> Add5/4
  alpha/1 -> Add5/1
  Subsystem1/1(Out1) -> Divide3/3
  Product5/1 -> Add5/3
  V/1 -> Subsystem1/1(In1)
  Constant12/1 -> Add5/2
  Constant14/1 -> Product5/2
  E/1 -> Add5/5
  q/1 -> Divide3/1

== system simulinkmodel/A//C/Subsystem20 ==
  note: Wing Lift Coefficient
  alpha : Inport
  Add : Sum
  Constant : Constant  Value=CLow
  Constant1 : Constant  Value=CLaw
  Product : Product
  CLw : Outport
  wires:
  alpha/1 -> Product/2
  Constant/1 -> Add/1
  Constant1/1 -> Product/1
  Product/1 -> Add/2
  Add/1 -> CLw/1  "CLw"

== system simulinkmodel/A//C/Subsystem21 ==
  note: Wing Drag Coefficient
  Kw : Inport
  CLw : Inport  Port=2
  Add1 : Sum
  Constant2 : Constant  Value=CDminw
  Math Function : Math  Operator=square
  Product2 : Product
  CDw : Outport
  wires:
  CLw/1 -> Math Function/1
  Math Function/1 -> Product2/2
  Constant2/1 -> Add1/1
  Product2/1 -> Add1/2
  Add1/1 -> CDw/1  "CLw"
  Kw/1 -> Product2/1

== system simulinkmodel/A//C/Subsystem22 ==
  note: Dynamic Pressure
  V : Inport
  Constant26 : Constant  Value=0.5
  Constant27 : Constant  Value=rho
  Math Function2 : Math  Operator=square
  Product10 : Product  Inputs=3
  qb : Outport
  wires:
  Math Function2/1 -> Product10/3
  Constant26/1 -> Product10/1
  V/1 -> Math Function2/1
  Constant27/1 -> Product10/2
  Product10/1 -> qb/1

== system simulinkmodel/A//C/Subsystem23 ==
  note: Wing Lift Force
  qb : Inport
  CLw : Inport  Port=2
  Constant28 : Constant  Value=S
  Product11 : Product  Inputs=3
  Lw : Outport
  wires:
  Constant28/1 -> Product11/2
  Product11/1 -> Lw/1
  CLw/1 -> Product11/3
  qb/1 -> Product11/1

== system simulinkmodel/A//C/Subsystem24 ==
  note: Wing Drag Force
  qb : Inport
  CDw : Inport  Port=2
  Constant29 : Constant  Value=S
  Product12 : Product  Inputs=3
  Dw : Outport
  wires:
  Constant29/1 -> Product12/2
  CDw/1 -> Product12/3
  Product12/1 -> Dw/1
  qb/1 -> Product12/1

== system simulinkmodel/A//C/Subsystem25 ==
  note: Aerodynamic Efficiency
  alpha : Inport
  alpha_dot : Inport  Port=2
  V : Inport  Port=3
  Add2 : Sum
  Add3 : Sum  Inputs=+-
  Add4 : Sum
  Constant10 : Constant  Value=CLaw
  Constant11 : Constant  Value=CLow
  Constant18 : Constant  Value=2
  Constant7 : Constant  Value=ARw
  Constant8 : Constant  Value=cgt
  Constant9 : Constant  Value=cgw
  Divide1 : Product  Inputs=**/
  Divide2 : Product  Inputs=**/
  Pi1 : Constant  Value=pi  OutDataTypeStr=Inherit: Inherit via back propagation
  Product3 : Product
  Product4 : Product
  Subsystem2 : Subsystem
  E : Outport
  wires:
  Divide1/1 -> E/1
  Add3/1 -> Product3/1
  Constant11/1 -> Add4/2
  alpha_dot/1 -> Divide2/1
  Constant18/1 -> Divide1/2
  Constant9/1 -> Add2/2
  Product3/1 -> Add4/1
  Constant8/1 -> Add2/1
  Divide2/1 -> Add3/2
  Constant10/1 -> Product3/2
  Product4/1 -> Divide1/3
  Add2/1 -> Divide2/2
  Add4/1 -> Divide1/1
  Pi1/1 -> Product4/1
  Constant7/1 -> Product4/2
  Subsystem2/1(Out1) -> Divide2/3
  alpha/1 -> Add3/1
  V/1 -> Subsystem2/1(In1)

== system simulinkmodel/A//C/Subsystem26 ==
  note: Wing Moments
  qb : Inport
  Constant30 : Constant  Value=S
  Constant31 : Constant  Value=c
  Constant32 : Constant  Value=Cmw
  Product13 : Product  Inputs=4
  Mw : Outport
  wires:
  qb/1 -> Product13/1
  Constant30/1 -> Product13/2
  Product13/1 -> Mw/1
  Constant31/1 -> Product13/3
  Constant32/1 -> Product13/4

== system simulinkmodel/A//C/Subsystem27 ==
  note: Fuselage Drag Force
  qb : Inport
  Constant37 : Constant  Value=S
  Constant38 : Constant  Value=CDf
  Product16 : Product  Inputs=3
  Df : Outport
  wires:
  Constant37/1 -> Product16/2
  Constant38/1 -> Product16/3
  qb/1 -> Product16/1
  Product16/1 -> Df/1

== system simulinkmodel/A//C/Subsystem28 ==
  note: Tail Lift Force
  qb : Inport
  CLt : Inport  Port=2
  Constant33 : Constant  Value=St
  Constant34 : Constant  Value=nt
  Product14 : Product  Inputs=4
  Lt : Outport
  wires:
  Constant34/1 -> Product14/1
  Constant33/1 -> Product14/3
  Product14/1 -> Lt/1
  qb/1 -> Product14/2
  CLt/1 -> Product14/4

== system simulinkmodel/A//C/Subsystem29 ==
  note: Tail Drag Force
  qb : Inport
  CDt : Inport  Port=2
  Constant35 : Constant  Value=nt
  Constant36 : Constant  Value=St
  Product15 : Product  Inputs=4
  Dt : Outport
  wires:
  Constant36/1 -> Product15/3
  Constant35/1 -> Product15/1
  qb/1 -> Product15/2
  Product15/1 -> Dt/1
  CDt/1 -> Product15/4

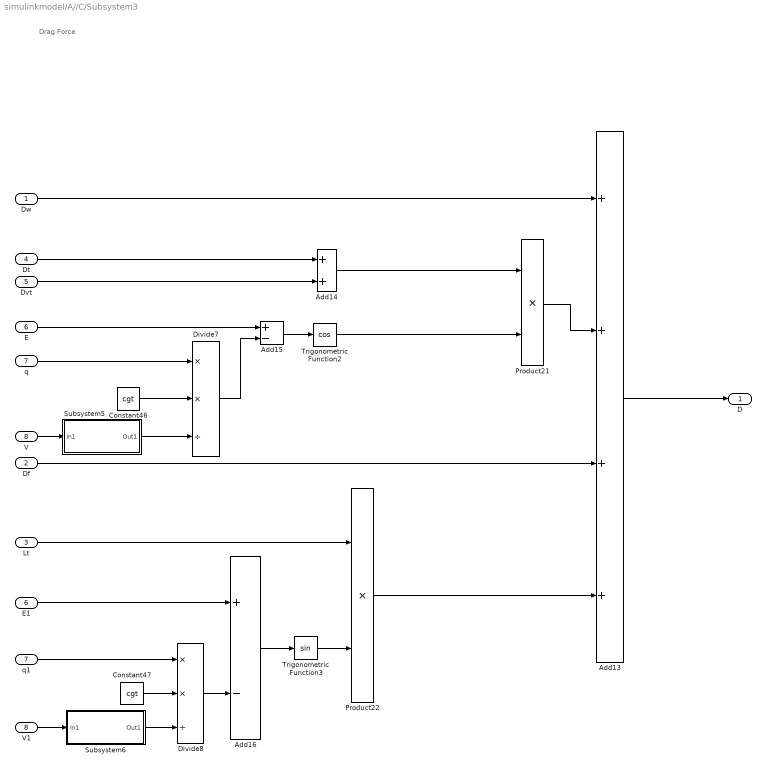
== system simulinkmodel/A//C/Subsystem3 ==
  note: Drag Force
  Dw : Inport
  Df : Inport  Port=2
  Lt : Inport  Port=3
  Dt : Inport  Port=4
  Dvt : Inport  Port=5
  E : Inport  Port=6
  q : Inport  Port=7
  V : Inport  Port=8
  Add13 : Sum  Inputs=++++
  Add14 : Sum
  Add15 : Sum  Inputs=+-
  Add16 : Sum  Inputs=+-
  Constant46 : Constant  Value=cgt
  Constant47 : Constant  Value=cgt
  Divide7 : Product  Inputs=**/
  Divide8 : Product  Inputs=**/
  E1 : InportShadow  Port=6
  Product21 : Product
  Product22 : Product
  Subsystem5 : Subsystem
  Subsystem6 : Subsystem
  Trigonometric Function2 : Trigonometry  Operator=cos
  Trigonometric Function3 : Trigonometry
  V1 : InportShadow  Port=8
  q1 : InportShadow  Port=7
  D : Outport
  wires:
  Add16/1 -> Trigonometric Function3/1
  Add15/1 -> Trigonometric Function2/1
  Add13/1 -> D/1
  Divide8/1 -> Add16/2
  Df/1 -> Add13/3
  Product21/1 -> Add13/2
  Lt/1 -> Product22/1
  Trigonometric Function2/1 -> Product21/2
  Constant47/1 -> Divide8/2
  Dvt/1 -> Add14/2
  Add14/1 -> Product21/1
  Divide7/1 -> Add15/2
  Product22/1 -> Add13/4
  Constant46/1 -> Divide7/2
  Subsystem6/1(Out1) -> Divide8/3
  Subsystem5/1(Out1) -> Divide7/3
  Trigonometric Function3/1 -> Product22/2
  E/1 -> Add15/1
  Dt/1 -> Add14/1
  q1/1 -> Divide8/1
  V1/1 -> Subsystem6/1(In1)
  E1/1 -> Add16/1
  Dw/1 -> Add13/1
  V/1 -> Subsystem5/1(In1)
  q/1 -> Divide7/1

== system simulinkmodel/A//C/Subsystem30 ==
  note: Fuselage Moments
  qb : Inport
  Cmf : Inport  Port=2
  Constant39 : Constant  Value=S
  Constant40 : Constant  Value=c
  Product17 : Product  Inputs=4
  Mf : Outport
  wires:
  Constant39/1 -> Product17/2
  Constant40/1 -> Product17/3
  Product17/1 -> Mf/1
  Cmf/1 -> Product17/4
  qb/1 -> Product17/1

== system simulinkmodel/A//C/Subsystem31 ==
  note: Vertical Tail Drag Force
  qb : Inport
  Constant41 : Constant  Value=nt
  Constant42 : Constant  Value=Svt
  Constant43 : Constant  Value=CDminvt
  Product18 : Product  Inputs=4
  Dvt : Outport
  wires:
  Constant43/1 -> Product18/4
  Constant41/1 -> Product18/1
  qb/1 -> Product18/2
  Product18/1 -> Dvt/1
  Constant42/1 -> Product18/3

== system simulinkmodel/A//C/Subsystem32 ==
  note: Rolling Moment Coefficient w.r.t Roll Rate
  Add7 : Sum
  Add8 : Sum
  Constant20 : Constant  Value=-1/12
  Constant21 : Constant  Value=CLaw
  Constant22 : Constant
  Constant23 : Constant
  Constant24 : Constant  Value=lambda
  Constant25 : Constant  Value=lambda
  Divide4 : Product  Inputs=*/
  Gain : Gain  Gain=3
  Product9 : Product  Inputs=3
  Clp : Outport
  wires:
  Divide4/1 -> Product9/3
  Constant21/1 -> Product9/2
  Constant25/1 -> Add8/2
  Constant22/1 -> Add7/1
  Add8/1 -> Divide4/2
  Constant20/1 -> Product9/1
  Constant24/1 -> Gain/1
  Constant23/1 -> Add8/1
  Gain/1 -> Add7/2
  Add7/1 -> Divide4/1
  Product9/1 -> Clp/1

== system simulinkmodel/A//C/Subsystem33 ==
  note: Fuselage Moment Coefficient
  alpha : Inport
  Constant19 : Constant  Value=Cmaf
  Product8 : Product
  Cmf : Outport
  wires:
  Constant19/1 -> Product8/1
  Product8/1 -> Cmf/1
  alpha/1 -> Product8/2

== system simulinkmodel/A//C/Subsystem34 ==
  note: Tail Drag Coefficient
  CLt : Inport
  Add6 : Sum
  Constant16 : Constant  Value=CDmint
  Constant17 : Constant  Value=Kt
  Math Function1 : Math  Operator=square
  Product7 : Product
  CDt : Outport
  wires:
  Constant16/1 -> Add6/1
  Constant17/1 -> Product7/1
  CLt/1 -> Math Function1/1
  Product7/1 -> Add6/2
  Add6/1 -> CDt/1
  Math Function1/1 -> Product7/2

== system simulinkmodel/A//C/Subsystem35 ==
  note: Lift Force
  Lw : Inport
  Lt : Inport  Port=2
  E : Inport  Port=3
  q : Inport  Port=4
  V : Inport  Port=5
  Dt : Inport  Port=6
  Dvt : Inport  Port=7
  In9 : Inport  Port=8
  In10 : Inport  Port=9
  Add10 : Sum  Inputs=+-
  Add11 : Sum
  Add12 : Sum  Inputs=+-
  Add9 : Sum  Inputs=++-
  Constant44 : Constant  Value=cgt
  Constant45 : Constant  Value=cgt
  Divide5 : Product  Inputs=**/
  Divide6 : Product  Inputs=**/
  E1 : InportShadow  Port=3
  Product19 : Product
  Product20 : Product
  Subsystem3 : Subsystem
  Subsystem4 : Subsystem
  Trigonometric Function : Trigonometry  Operator=cos
  Trigonometric Function1 : Trigonometry
  L : Outport
  wires:
  Product19/1 -> Add9/2
  Add11/1 -> Product20/1
  Lt/1 -> Product19/1
  Add12/1 -> Trigonometric Function1/1
  Add10/1 -> Trigonometric Function/1
  Subsystem3/1(Out1) -> Divide6/3
  Constant44/1 -> Divide5/2
  Divide5/1 -> Add10/2
  Divide6/1 -> Add12/2
  Trigonometric Function1/1 -> Product20/2
  Product20/1 -> Add9/3
  Dvt/1 -> Add11/2
  Constant45/1 -> Divide6/2
  Trigonometric Function/1 -> Product19/2
  E1/1 -> Add12/1
  Subsystem4/1(Out1) -> Divide5/3
  Dt/1 -> Add11/1
  Lw/1 -> Add9/1
  Add9/1 -> L/1
  In10/1 -> Subsystem3/1(In1)
  V/1 -> Subsystem4/1(In1)
  q/1 -> Divide5/1
  E/1 -> Add10/1
  In9/1 -> Divide6/1

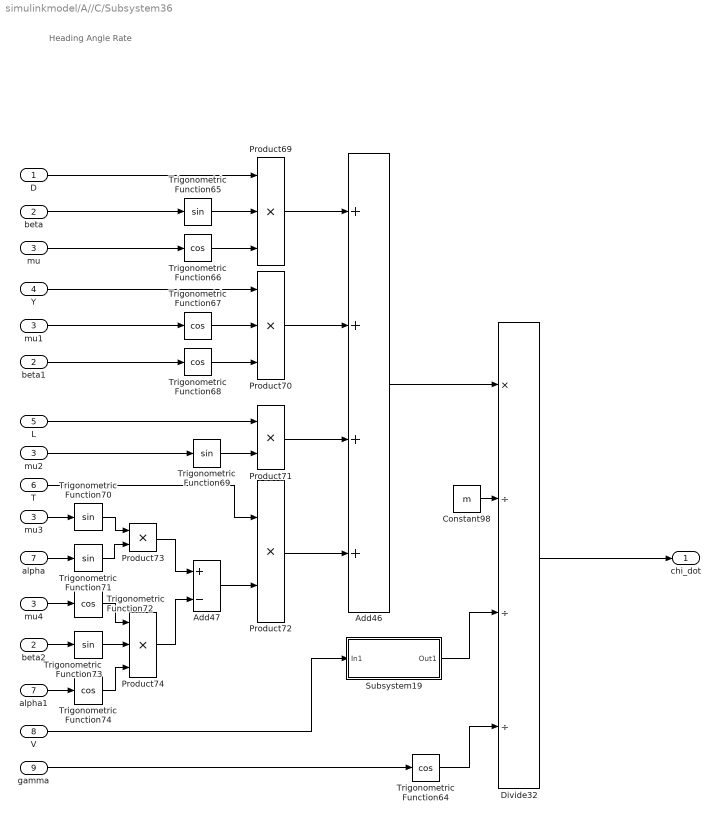
== system simulinkmodel/A//C/Subsystem36 ==
  note: Heading Angle Rate
  D : Inport
  beta : Inport  Port=2
  mu : Inport  Port=3
  Y : Inport  Port=4
  L : Inport  Port=5
  T : Inport  Port=6
  alpha : Inport  Port=7
  V : Inport  Port=8
  gamma : Inport  Port=9
  Add46 : Sum  Inputs=++++
  Add47 : Sum  Inputs=+-
  Constant98 : Constant  Value=m
  Divide32 : Product  Inputs=*///
  Product69 : Product  Inputs=3
  Product70 : Product  Inputs=3
  Product71 : Product
  Product72 : Product
  Product73 : Product
  Product74 : Product  Inputs=3
  Subsystem19 : Subsystem
  Trigonometric Function{64,66..68,72,74} (6 alike) : Trigonometry  Operator=cos
  Trigonometric Function{65,69..71,73} (5 alike) : Trigonometry
  alpha1 : InportShadow  Port=7
  beta1 : InportShadow  Port=2
  beta2 : InportShadow  Port=2
  mu{1..4} (4 alike) : InportShadow  Port=3
  chi_dot : Outport
  wires:
  Product70/1 -> Add46/2
  Product73/1 -> Add47/1
  Trigonometric Function69/1 -> Product71/2
  Trigonometric Function67/1 -> Product70/2
  Product74/1 -> Add47/2
  Subsystem19/1(Out1) -> Divide32/3
  L/1 -> Product71/1
  mu1/1 -> Trigonometric Function67/1
  Product71/1 -> Add46/3
  Divide32/1 -> chi_dot/1
  Trigonometric Function73/1 -> Product74/2
  beta1/1 -> Trigonometric Function68/1
  alpha1/1 -> Trigonometric Function74/1
  Trigonometric Function71/1 -> Product73/2
  V/1 -> Subsystem19/1(In1)
  Trigonometric Function70/1 -> Product73/1
  Trigonometric Function72/1 -> Product74/1
  Trigonometric Function66/1 -> Product69/3
  alpha/1 -> Trigonometric Function71/1
  mu2/1 -> Trigonometric Function69/1
  Constant98/1 -> Divide32/2
  Trigonometric Function64/1 -> Divide32/4
  gamma/1 -> Trigonometric Function64/1
  Trigonometric Function68/1 -> Product70/3
  beta/1 -> Trigonometric Function65/1
  mu4/1 -> Trigonometric Function72/1
  Trigonometric Function65/1 -> Product69/2
  mu/1 -> Trigonometric Function66/1
  Trigonometric Function74/1 -> Product74/3
  Product69/1 -> Add46/1
  Product72/1 -> Add46/4
  Add46/1 -> Divide32/1
  Add47/1 -> Product72/2
  mu3/1 -> Trigonometric Function70/1
  T/1 -> Product72/1
  D/1 -> Product69/1
  Y/1 -> Product70/1
  beta2/1 -> Trigonometric Function73/1

== system simulinkmodel/A//C/Subsystem4 ==
  note: Side Force
  qb : Inport
  beta : Inport  Port=2
  drt : Inport  Port=3
  r : Inport  Port=4
  V : Inport  Port=5
  Add17 : Sum  Inputs=-++
  Constant48 : Constant  Value=nvt
  Constant49 : Constant  Value=Svt
  Constant50 : Constant  Value=CLavt
  Constant51 : Constant  Value=Tr
  Constant52 : Constant  Value=cgvt
  Divide9 : Product  Inputs=**/
  Product23 : Product  Inputs=5
  Product24 : Product
  Subsystem7 : Subsystem
  Y : Outport
  wires:
  Constant49/1 -> Product23/3
  Constant50/1 -> Product23/4
  Constant48/1 -> Product23/1
  Product24/1 -> Add17/2
  Constant52/1 -> Divide9/2
  Constant51/1 -> Product24/1
  Subsystem7/1(Out1) -> Divide9/3
  Add17/1 -> Product23/5
  Product23/1 -> Y/1
  Divide9/1 -> Add17/3
  V/1 -> Subsystem7/1(In1)
  beta/1 -> Add17/1
  qb/1 -> Product23/2
  drt/1 -> Product24/2
  r/1 -> Divide9/1

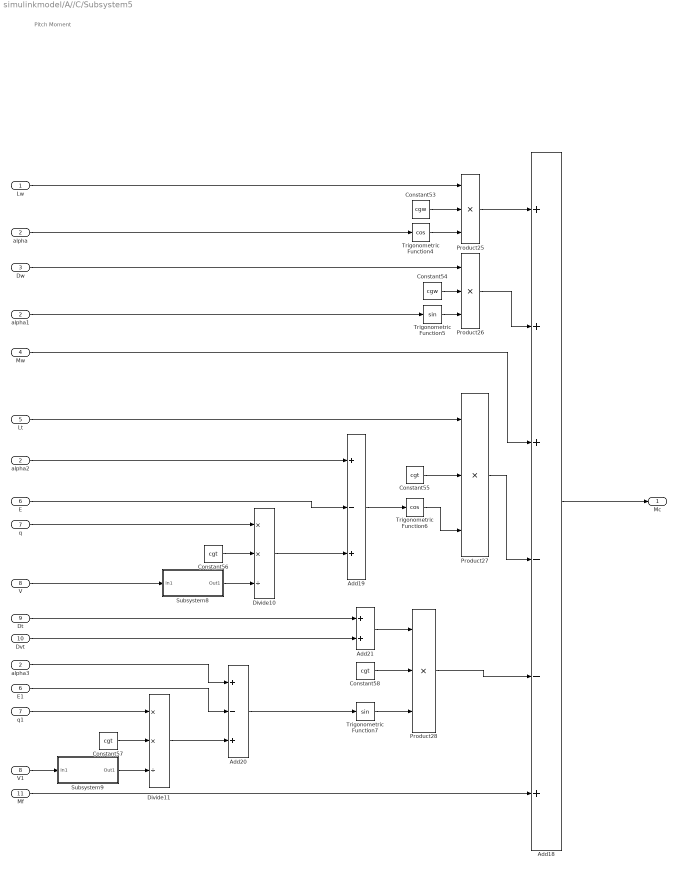
== system simulinkmodel/A//C/Subsystem5 ==
  note: Pitch Moment
  Lw : Inport
  alpha : Inport  Port=2
  Dw : Inport  Port=3
  Mw : Inport  Port=4
  Lt : Inport  Port=5
  E : Inport  Port=6
  q : Inport  Port=7
  V : Inport  Port=8
  Dt : Inport  Port=9
  Dvt : Inport  Port=10
  Mf : Inport  Port=11
  Add18 : Sum  Inputs=+++--+
  Add19 : Sum  Inputs=+-+
  Add20 : Sum  Inputs=+-+
  Add21 : Sum
  Constant53 : Constant  Value=cgw
  Constant54 : Constant  Value=cgw
  Constant{55..58} (4 alike) : Constant  Value=cgt
  Divide10 : Product  Inputs=**/
  Divide11 : Product  Inputs=**/
  E1 : InportShadow  Port=6
  Product{25..28} (4 alike) : Product  Inputs=3
  Subsystem8 : Subsystem
  Subsystem9 : Subsystem
  Trigonometric Function4 : Trigonometry  Operator=cos
  Trigonometric Function5 : Trigonometry
  Trigonometric Function6 : Trigonometry  Operator=cos
  Trigonometric Function7 : Trigonometry
  V1 : InportShadow  Port=8
  alpha1 : InportShadow  Port=2
  alpha2 : InportShadow  Port=2
  alpha3 : InportShadow  Port=2
  q1 : InportShadow  Port=7
  Mc : Outport
  wires:
  Constant54/1 -> Product26/2
  Product25/1 -> Add18/1
  alpha/1 -> Trigonometric Function4/1
  Subsystem8/1(Out1) -> Divide10/3
  Add20/1 -> Trigonometric Function7/1
  Constant53/1 -> Product25/2
  Divide11/1 -> Add20/3
  Constant58/1 -> Product28/2
  Trigonometric Function5/1 -> Product26/3
  V/1 -> Subsystem8/1(In1)
  Trigonometric Function6/1 -> Product27/3
  Divide10/1 -> Add19/3
  Product27/1 -> Add18/4
  E/1 -> Add19/2
  Constant55/1 -> Product27/2
  Dw/1 -> Product26/1
  Lw/1 -> Product25/1
  Trigonometric Function7/1 -> Product28/3
  Product26/1 -> Add18/2
  Add21/1 -> Product28/1
  q/1 -> Divide10/1
  Trigonometric Function4/1 -> Product25/3
  Mw/1 -> Add18/3
  Constant56/1 -> Divide10/2
  Subsystem9/1(Out1) -> Divide11/3
  Add19/1 -> Trigonometric Function6/1
  Product28/1 -> Add18/5
  Constant57/1 -> Divide11/2
  Mf/1 -> Add18/6
  q1/1 -> Divide11/1
  Dt/1 -> Add21/1
  Lt/1 -> Product27/1
  Add18/1 -> Mc/1
  E1/1 -> Add20/2
  V1/1 -> Subsystem9/1(In1)
  alpha1/1 -> Trigonometric Function5/1
  alpha2/1 -> Add19/1
  Dvt/1 -> Add21/2
  alpha3/1 -> Add20/1

== system simulinkmodel/A//C/Subsystem6 ==
  note: Yaw Moment
  qb : Inport
  beta : Inport  Port=2
  drt : Inport  Port=3
  r : Inport  Port=4
  V : Inport  Port=5
  da : Inport  Port=6
  Add22 : Sum  Inputs=--
  Add23 : Sum  Inputs=-++
  Constant59 : Constant  Value=nvt
  Constant60 : Constant  Value=Svt
  Constant61 : Constant  Value=CLavt
  Constant62 : Constant  Value=cgvt
  Constant63 : Constant  Value=Tr
  Constant64 : Constant  Value=cgvt
  Constant65 : Constant  Value=S
  Constant66 : Constant  Value=b
  Constant67 : Constant  Value=Cnda
  Divide12 : Product  Inputs=**/
  Product29 : Product  Inputs=6
  Product30 : Product
  Product31 : Product  Inputs=5
  Subsystem10 : Subsystem
  qb1 : InportShadow
  Nc : Outport
  wires:
  Subsystem10/1(Out1) -> Divide12/3
  Constant63/1 -> Product30/1
  Constant65/1 -> Product31/2
  Constant62/1 -> Product29/6
  drt/1 -> Product30/2
  Constant61/1 -> Product29/4
  Product30/1 -> Add23/2
  qb1/1 -> Product31/1
  Add23/1 -> Product29/5
  Constant59/1 -> Product29/2
  Constant64/1 -> Divide12/2
  Constant60/1 -> Product29/3
  Product29/1 -> Add22/1
  Divide12/1 -> Add23/3
  Product31/1 -> Add22/2
  Constant67/1 -> Product31/4
  Constant66/1 -> Product31/3
  Add22/1 -> Nc/1
  r/1 -> Divide12/1
  qb/1 -> Product29/1
  da/1 -> Product31/5
  beta/1 -> Add23/1
  V/1 -> Subsystem10/1(In1)
